simulink model "Pendulum_ClosedLoop_Reference"  (R2023a)
settings: Solver=ode4  StartTime=0.0  StopTime=5  FixedStep=0.001  RelTol=1e-3
settings Model: Creator=Fasih  LastModifiedBy=Fasih

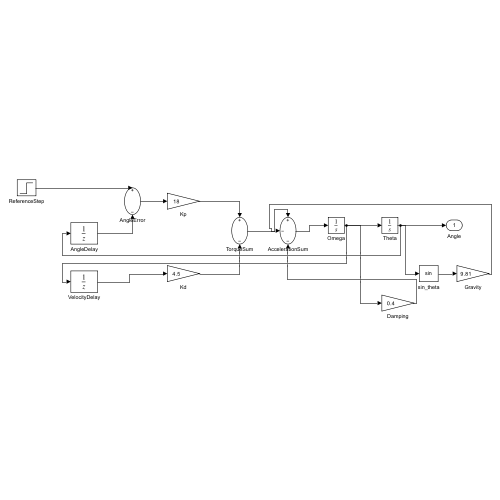
[thumbnail: Simulink's stored preview of the top-level diagram]
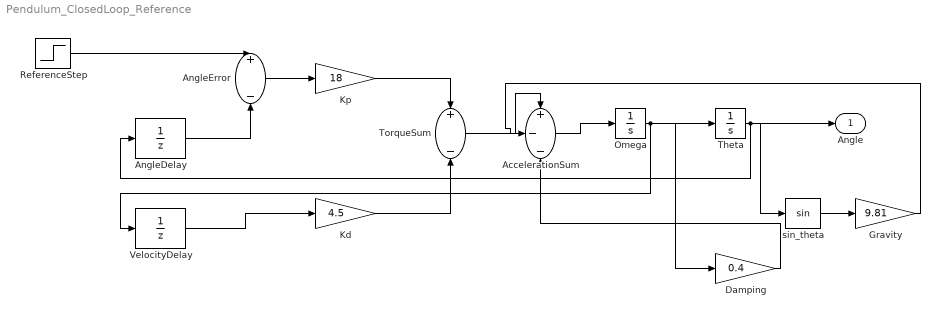
== system Pendulum_ClosedLoop_Reference ==
  AccelerationSum : Sum  Inputs=+--
  AngleDelay : UnitDelay  SampleTime=0.001  HasFrameUpgradeWarning=on
  AngleError : Sum  Inputs=+-
  Damping : Gain  Gain=0.4
  Gravity : Gain  Gain=9.81
  Kd : Gain  Gain=4.5
  Kp : Gain  Gain=18
  Omega : Integrator
  ReferenceStep : Step  Time=0  After=0.4  SampleTime=0
  Theta : Integrator
  TorqueSum : Sum  Inputs=+-
  VelocityDelay : UnitDelay  SampleTime=0.001  HasFrameUpgradeWarning=on
  sin_theta : Trigonometry
  Angle : Outport
  wires:
  ReferenceStep/1 -> AngleError/1
  AngleDelay/1 -> AngleError/2
  AngleError/1 -> Kp/1
  VelocityDelay/1 -> Kd/1
  Kp/1 -> TorqueSum/1
  Kd/1 -> TorqueSum/2
  TorqueSum/1 -> AccelerationSum/1
  AccelerationSum/1 -> Omega/1
  Omega/1 -> Theta/1, VelocityDelay/1, Damping/1
  Theta/1 -> Angle/1, AngleDelay/1, sin_theta/1
  sin_theta/1 -> Gravity/1
  Gravity/1 -> AccelerationSum/2
  Damping/1 -> AccelerationSum/3
